simulink model "Tut14_AtomicSubsystem_Part2"  (R2021a)
settings: Solver=FixedStepDiscrete  StartTime=0.0  StopTime=10.0  FixedStep=1  RelTol=1e-3
settings Model: Creator=cheta  LastModifiedBy=cheta
settings OptimizationCC: DefaultParameterBehavior=Inlined  EnhancedBackFolding=on  PassReuseOutputArgsAs=Individual arguments  ZeroExternalMemoryAtStartup=off  ZeroInternalMemoryAtStartup=off  OptimizeBlockOrder=speed  DifferentSizesBufferReuse=on  OptimizationCustomize=off  EfficientTunableParamExpr=on
settings DebuggingCC: ParameterTunabilityLossMsg=error
settings SFSimCC: MATLABDynamicMemAlloc=off
settings RTWCC: SystemTargetFile=ert.tlc  TemplateMakefile=ert_default_tmf
settings CodeAppCC: ForceParamTrailComments=on  IgnoreCustomStorageClasses=off  OperatorAnnotations=on  SimulinkDataObjDesc=on  SFDataObjDesc=on  InsertBlockDesc=on
settings ERTTargetCC: TargetLangStandard=C99 (ISO)  GenerateSampleERTMain=on  InlinedParameterPlacement=NonHierarchical  ERTCustomFileTemplate=example_file_process.tlc

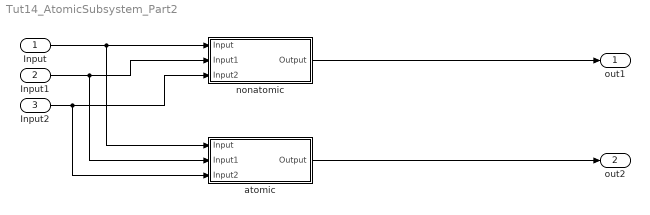
== system Tut14_AtomicSubsystem_Part2 ==
  Input : Inport
  Input1 : Inport  Port=2
  Input2 : Inport  Port=3
  atomic : Subsystem  TreatAsAtomicUnit=on
      settings: FunctionWithSeparateData=on
  nonatomic : Subsystem
  out1 : Outport
  out2 : Outport  Port=2
  wires:
  nonatomic/1(Output) -> out1/1
  Input/1 -> atomic/1(Input), nonatomic/1(Input)
  Input1/1 -> atomic/2(Input1), nonatomic/2(Input1)
  Input2/1 -> atomic/3(Input2), nonatomic/3(Input2)
  atomic/1(Output) -> out2/1

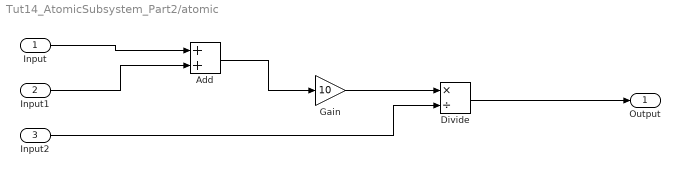
== system Tut14_AtomicSubsystem_Part2/atomic ==
  Input : Inport
  Input1 : Inport  Port=2
  Input2 : Inport  Port=3
  Add : Sum
  Divide : Product  Inputs=*/
  Gain : Gain  Gain=10
  Output : Outport
  wires:
  Divide/1 -> Output/1
  Input2/1 -> Divide/2
  Gain/1 -> Divide/1
  Add/1 -> Gain/1
  Input1/1 -> Add/2
  Input/1 -> Add/1

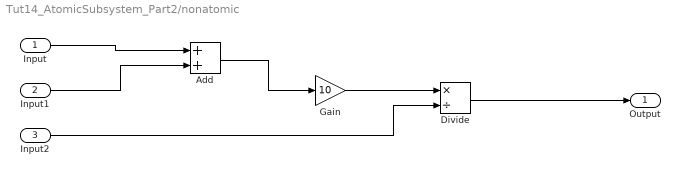
== system Tut14_AtomicSubsystem_Part2/nonatomic ==
  Input : Inport
  Input1 : Inport  Port=2
  Input2 : Inport  Port=3
  Add : Sum
  Divide : Product  Inputs=*/
  Gain : Gain  Gain=10
  Output : Outport
  wires:
  Input/1 -> Add/1
  Input1/1 -> Add/2
  Add/1 -> Gain/1
  Gain/1 -> Divide/1
  Input2/1 -> Divide/2
  Divide/1 -> Output/1
